simulink model "TEST"  (R2020b)
settings: Solver=VariableStepAuto  StartTime=0.0  StopTime=10.0  MaxStep=1e-4  RelTol=1e-3
undefined symbols (not defined in the file): b, g, I, l, m, M
settings Model: Creator=sansh  LastModifiedBy=ricardo
settings DataIOCC: ReturnWorkspaceOutputs=off
settings DebuggingCC: ArithmeticOperatorsInVariantConditions=warning
settings SFSimCC: SimUseLocalCustomCode=off  CustomCodeUndefinedFunction=UseInterfaceOnly
settings RTWCC: RTWUseLocalCustomCode=off
settings CodeAppCC: StateflowObjectComments=on

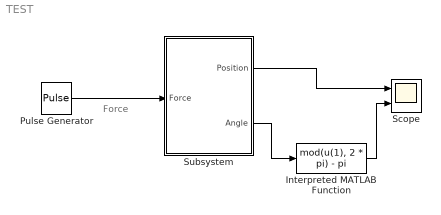
== system TEST ==
  note: Force
  Interpreted MATLAB Function : MATLABFcn  MATLABFcn=mod(u(1), 2 * pi) - pi
  Pulse Generator : DiscretePulseGenerator  PulseType=Time based  Amplitude=1000  Period=10  PulseWidth=0.01
  Scope : Scope  NumInputPorts=2
  Subsystem : Subsystem
  wires:
  Pulse Generator/1 -> Subsystem/1(Force)
  Subsystem/1(Position) -> Scope/1
  Subsystem/2(Angle) -> Interpreted MATLAB Function/1
  Interpreted MATLAB Function/1 -> Scope/2

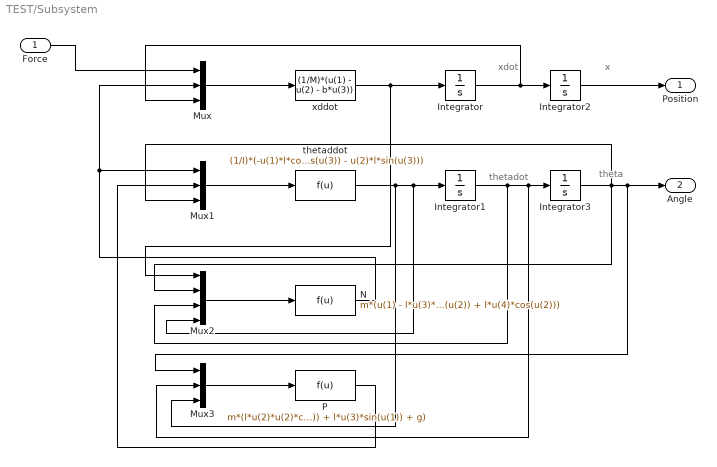
== system TEST/Subsystem ==
  note: theta
  note: x
  note: thetadot
  note: xdot
  Force : Inport
  Integrator : Integrator  ContinuousStateAttributes='xdot'
  Integrator1 : Integrator  ContinuousStateAttributes='thetadot'
  Integrator2 : Integrator  ContinuousStateAttributes='x'
  Integrator3 : Integrator  InitialCondition=pi  ContinuousStateAttributes='theta'
  Mux : Mux  Inputs=3
  Mux1 : Mux  Inputs=3
  Mux2 : Mux
  Mux3 : Mux  Inputs=3
  N : Fcn  Expr=m*(u(1) - l*u(3)*u(3)*sin(u(2)) + l*u(4)*cos(u(2)))
  P : Fcn  Expr=m*(l*u(2)*u(2)*cos(u(1)) + l*u(3)*sin(u(1)) + g)
  thetaddot : Fcn  Expr=(1/I)*(-u(1)*l*cos(u(3)) - u(2)*l*sin(u(3)))
  xddot : Fcn  Expr=(1/M)*(u(1) - u(2) - b*u(3))
  Position : Outport
  Angle : Outport  Port=2
  wires:
  Force/1 -> Mux/1
  Mux2/1 -> N/1
  Mux/1 -> xddot/1
  P/1 -> Mux1/2
  Mux3/1 -> P/1
  N/1 -> Mux1/1, Mux/2
  Mux1/1 -> thetaddot/1
  xddot/1 -> Mux2/1, Integrator/1
  Integrator2/1 -> Position/1
  thetaddot/1 -> Mux3/3, Mux2/4, Integrator1/1
  Integrator/1 -> Mux/3, Integrator2/1
  Integrator1/1 -> Mux2/3, Mux3/2, Integrator3/1
  Integrator3/1 -> Mux2/2, Mux1/3, Angle/1, Mux3/1
